simulink model "Control_no_lineal_cartesiano_2018b_charlo"  (R2018b)
settings: Solver=VariableStepAuto  StartTime=0.0  StopTime=15  RelTol=1e-3
PreLoadFcn:
  | AUT_TP1_1;
InitFcn:
  | AUT_TP1_1;
undefined symbols (not defined in the file or in its folder): cfg
libraries: roblocks x2, simulink x1
settings Model: Creator=Acer  LastModifiedBy=Carlos
settings DataIOCC: ReturnWorkspaceOutputs=on
settings DebuggingCC: SFMachineParentedDataDiag=error

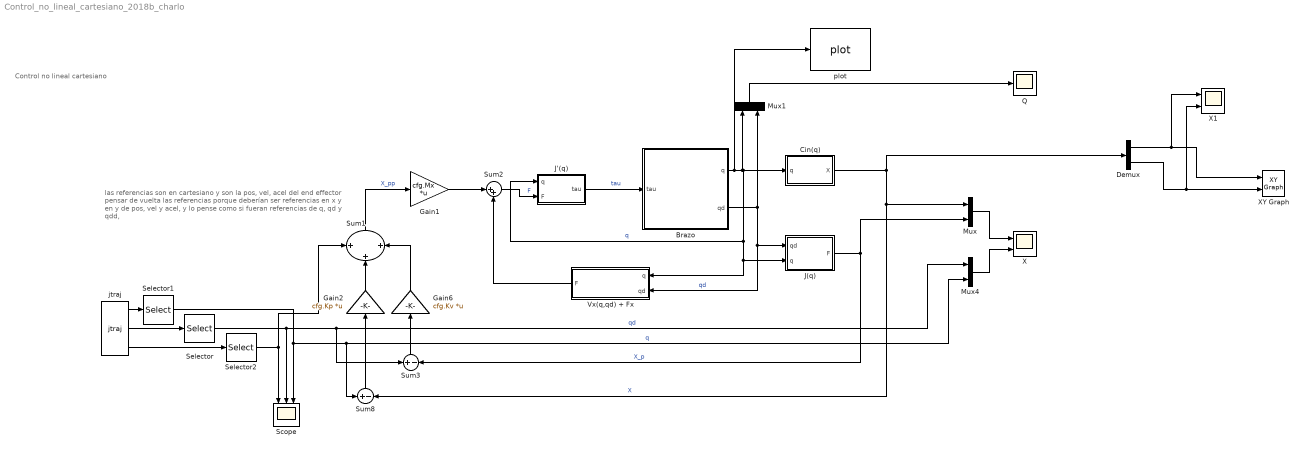
== system Control_no_lineal_cartesiano_2018b_charlo ==
  note: las referencias son en cartesiano
      | y son la pos, vel, acel del end effector
      |
      | pensar de vuelta las referencias porque deberían ser
      | referencias en x y en y de pos, vel y acel, y lo pense como si fueran
      | referencias de q, qd y qdd,
  note: Control no lineal cartesiano
  Brazo : Subsystem
      mask Display: image('brazo.jpg')
  Cin(q) : Subsystem
  Demux : Demux  Outputs=2
  Gain1 : Gain  Gain=cfg.Mx  Multiplication=Matrix(K*u) (u vector)
  Gain2 : Gain  Gain=cfg.Kp  Multiplication=Matrix(K*u) (u vector)
  Gain6 : Gain  Gain=cfg.Kv  Multiplication=Matrix(K*u) (u vector)
  J'(q) : Subsystem
  J(q) : Subsystem
  Mux : Mux  Inputs=2
  Mux1 : Mux  Inputs=2
  Mux4 : Mux  Inputs=2
  Q : Scope
  Scope : Scope  NumInputPorts=3
  Selector : Selector  InputPortWidth=6  IndexOptions=Index vector (dialog)  Indices=[1 2]  OutputSizes=1
  Selector1 : Selector  InputPortWidth=6  IndexOptions=Index vector (dialog)  Indices=[1 2]  OutputSizes=1
  Selector2 : Selector  InputPortWidth=6  IndexOptions=Index vector (dialog)  Indices=[1 2]  OutputSizes=1
  Sum1 : Sum  Inputs=+|+|+
  Sum2 : Sum  Inputs=|++
  Sum3 : Sum  Inputs=+-
  Sum8 : Sum  Inputs=+-
  Vx(q,qd) + Fx : Subsystem
  X : Scope  NumInputPorts=2
  X1 : Scope  NumInputPorts=2
  XY Graph : simulink/Sinks/XY Graph  xmin=-2  xmax=2  ymin=-2  ymax=2  st=-1
  jtraj : roblocks/Toolbox/jtraj  q0=[1 -1 0 0 0 0]  qf=[1 1 0 0 0 0]  tmax=2  ts=0.02
  plot : roblocks/Arm/plot  robot=messi  fps=10  holdplot=on
  wires:
  Sum1/1 -> Gain1/1  "X_pp"
  Sum3/1 -> Gain6/1
  Sum8/1 -> Gain2/1
  Gain6/1 -> Sum1/3
  Gain1/1 -> Sum2/1
  Gain2/1 -> Sum1/2
  Sum2/1 -> J'(q)/1(F)  "F"
  J'(q)/1(tau) -> Brazo/1(tau)  "tau"
  Brazo/2(qd) -> Vx(q,qd) + Fx/2(qd), J(q)/1(qd), Mux1/2  "qd"
  J(q)/1(F) -> Mux/2, Sum3/2  "X_p"
  Cin(q)/1(X) -> Mux/1, Sum8/2, Demux/1  "X"
  Vx(q,qd) + Fx/1(F) -> Sum2/2
  Brazo/1(q) -> plot/1, Cin(q)/1(q), J(q)/2(q), Vx(q,qd) + Fx/1(q), J'(q)/2(q), Mux1/1  "q"
  Mux/1 -> X/1
  Mux1/1 -> Q/1
  jtraj/1 -> Selector1/1
  jtraj/2 -> Selector/1
  Mux4/1 -> X/2
  jtraj/3 -> Selector2/1
  Selector/1 -> Mux4/1, Sum3/1, Scope/2  "qd"
  Selector1/1 -> Mux4/2, Sum8/1, Scope/3  "q"
  Selector2/1 -> Sum1/1, Scope/1
  Demux/1 -> X1/1, XY Graph/1
  Demux/2 -> X1/2, XY Graph/2

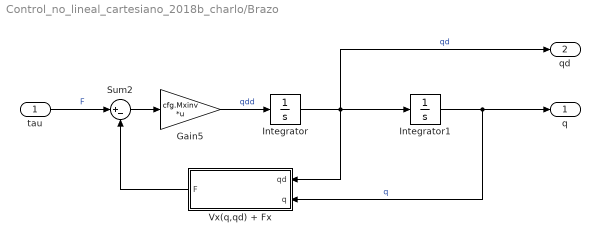
== system Control_no_lineal_cartesiano_2018b_charlo/Brazo ==
  tau : Inport
  Gain5 : Gain  Gain=cfg.Mxinv  Multiplication=Matrix(K*u) (u vector)
  Integrator : Integrator  InitialCondition=[0 0]
  Integrator1 : Integrator  InitialCondition=[0 -pi/2]
  Sum2 : Sum  Inputs=|+-
  Vx(q,qd) + Fx : Subsystem
  q : Outport  VectorParamsAs1DForOutWhenUnconnected=on
  qd : Outport  Port=2  VectorParamsAs1DForOutWhenUnconnected=on
  wires:
  Gain5/1 -> Integrator/1  "qdd"
  Integrator/1 -> Vx(q,qd) + Fx/1(qd), Integrator1/1, qd/1  "qd"
  tau/1 -> Sum2/1  "F"
  Sum2/1 -> Gain5/1
  Integrator1/1 -> Vx(q,qd) + Fx/2(q), q/1  "q"
  Vx(q,qd) + Fx/1(F) -> Sum2/2

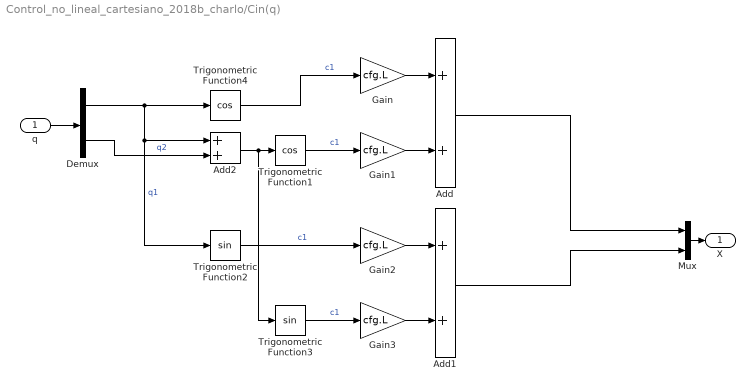
== system Control_no_lineal_cartesiano_2018b_charlo/Cin(q) ==
  q : Inport
  Add : Sum
  Add1 : Sum
  Add2 : Sum
  Demux : Demux  Outputs=2
  Gain{,1..3} (4 alike) : Gain  Gain=cfg.L
  Mux : Mux  Inputs=2
  Trigonometric Function1 : Trigonometry  Operator=cos
  Trigonometric Function2 : Trigonometry
  Trigonometric Function3 : Trigonometry
  Trigonometric Function4 : Trigonometry  Operator=cos
  X : Outport  VectorParamsAs1DForOutWhenUnconnected=on
  wires:
  Demux/1 -> Trigonometric Function2/1, Add2/1, Trigonometric Function4/1  "q1"
  q/1 -> Demux/1
  Mux/1 -> X/1
  Trigonometric Function4/1 -> Gain/1  "c1"
  Gain/1 -> Add/1
  Demux/2 -> Add2/2  "q2"
  Add2/1 -> Trigonometric Function3/1, Trigonometric Function1/1
  Trigonometric Function1/1 -> Gain1/1  "c1"
  Add/1 -> Mux/1
  Gain1/1 -> Add/2
  Trigonometric Function2/1 -> Gain2/1  "c1"
  Gain2/1 -> Add1/1
  Gain3/1 -> Add1/2
  Trigonometric Function3/1 -> Gain3/1  "c1"
  Add1/1 -> Mux/2

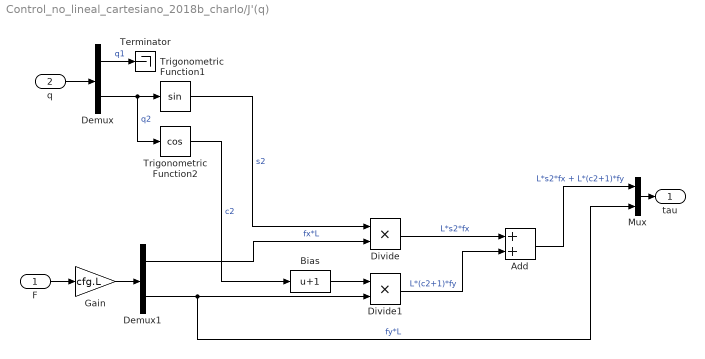
== system Control_no_lineal_cartesiano_2018b_charlo/J'(q) ==
  F : Inport
  q : Inport  Port=2
  Add : Sum
  Bias : Bias  Bias=1
  Demux : Demux  Outputs=2
  Demux1 : Demux  Outputs=2
  Divide : Product  Inputs=**
  Divide1 : Product  Inputs=**
  Gain : Gain  Gain=cfg.L
  Mux : Mux  Inputs=2
  Terminator : Terminator
  Trigonometric Function1 : Trigonometry
  Trigonometric Function2 : Trigonometry  Operator=cos
  tau : Outport  VectorParamsAs1DForOutWhenUnconnected=on
  wires:
  Demux/2 -> Trigonometric Function2/1, Trigonometric Function1/1  "q2"
  Demux/1 -> Terminator/1  "q1"
  q/1 -> Demux/1
  Trigonometric Function1/1 -> Divide/1  "s2"
  Trigonometric Function2/1 -> Bias/1  "c2"
  Demux1/1 -> Divide/2  "fx*L"
  Demux1/2 -> Mux/2, Divide1/2  "fy*L"
  Mux/1 -> tau/1
  F/1 -> Gain/1
  Gain/1 -> Demux1/1
  Divide/1 -> Add/1  "L*s2*fx"
  Bias/1 -> Divide1/1
  Divide1/1 -> Add/2  "L*(c2+1)*fy"
  Add/1 -> Mux/1  "L*s2*fx + L*(c2+1)*fy"

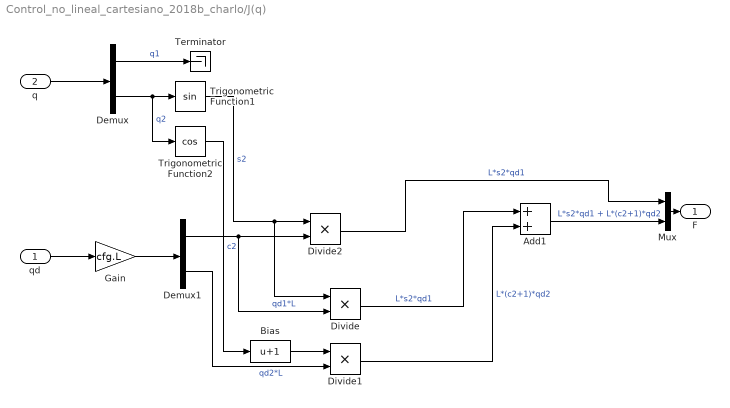
== system Control_no_lineal_cartesiano_2018b_charlo/J(q) ==
  qd : Inport
  q : Inport  Port=2
  Add1 : Sum
  Bias : Bias  Bias=1
  Demux : Demux  Outputs=2
  Demux1 : Demux  Outputs=2
  Divide : Product  Inputs=**
  Divide1 : Product  Inputs=**
  Divide2 : Product  Inputs=**
  Gain : Gain  Gain=cfg.L
  Mux : Mux  Inputs=2
  Terminator : Terminator
  Trigonometric Function1 : Trigonometry
  Trigonometric Function2 : Trigonometry  Operator=cos
  F : Outport  VectorParamsAs1DForOutWhenUnconnected=on
  wires:
  Divide1/1 -> Add1/2  "L*(c2+1)*qd2"
  Divide/1 -> Add1/1  "L*s2*qd1"
  q/1 -> Demux/1
  Bias/1 -> Divide1/1
  Demux/2 -> Trigonometric Function2/1, Trigonometric Function1/1  "q2"
  Gain/1 -> Demux1/1
  Mux/1 -> F/1
  Demux/1 -> Terminator/1  "q1"
  qd/1 -> Gain/1
  Add1/1 -> Mux/2  "L*s2*qd1 + L*(c2+1)*qd2"
  Demux1/1 -> Divide/2, Divide2/2  "qd1*L"
  Trigonometric Function1/1 -> Divide/1, Divide2/1  "s2"
  Divide2/1 -> Mux/1  "L*s2*qd1"
  Demux1/2 -> Divide1/2  "qd2*L"
  Trigonometric Function2/1 -> Bias/1  "c2"

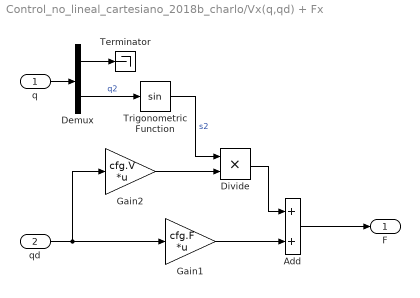
== system Control_no_lineal_cartesiano_2018b_charlo/Vx(q,qd) + Fx ==
  q : Inport
  qd : Inport  Port=2
  Add : Sum
  Demux : Demux  Outputs=2
  Divide : Product  Inputs=**
  Gain1 : Gain  Gain=cfg.F  Multiplication=Matrix(K*u) (u vector)
  Gain2 : Gain  Gain=cfg.V  Multiplication=Matrix(K*u) (u vector)
  Terminator : Terminator
  Trigonometric Function : Trigonometry
  F : Outport  VectorParamsAs1DForOutWhenUnconnected=on
  wires:
  qd/1 -> Gain1/1, Gain2/1
  Gain1/1 -> Add/2
  Add/1 -> F/1
  Gain2/1 -> Divide/2
  q/1 -> Demux/1
  Demux/1 -> Terminator/1
  Demux/2 -> Trigonometric Function/1  "q2"
  Divide/1 -> Add/1
  Trigonometric Function/1 -> Divide/1  "s2"

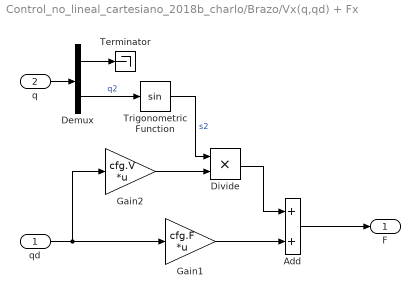
== system Control_no_lineal_cartesiano_2018b_charlo/Brazo/Vx(q,qd) + Fx ==
  qd : Inport
  q : Inport  Port=2
  Add : Sum
  Demux : Demux  Outputs=2
  Divide : Product  Inputs=**
  Gain1 : Gain  Gain=cfg.F  Multiplication=Matrix(K*u) (u vector)
  Gain2 : Gain  Gain=cfg.V  Multiplication=Matrix(K*u) (u vector)
  Terminator : Terminator
  Trigonometric Function : Trigonometry
  F : Outport  VectorParamsAs1DForOutWhenUnconnected=on
  wires:
  qd/1 -> Gain1/1, Gain2/1
  Gain1/1 -> Add/2
  Add/1 -> F/1
  Gain2/1 -> Divide/2
  q/1 -> Demux/1
  Demux/1 -> Terminator/1
  Demux/2 -> Trigonometric Function/1  "q2"
  Divide/1 -> Add/1
  Trigonometric Function/1 -> Divide/1  "s2"
